simulink model "test_motor_2016a"  (R2016a)
settings: Solver=ode45  StartTime=0.0  StopTime=0.5  RelTol=1e-3
settings Model: Creator=Matias  LastModifiedBy=tomej
settings DataIOCC: SaveFormat=Structure

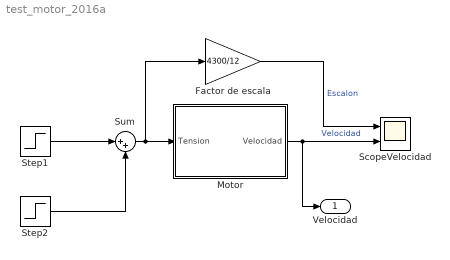
== system test_motor_2016a ==
  Factor de escala : Gain  Gain=4300/12
  Motor : Subsystem
  ScopeVelocidad : Scope  NumInputPorts=2
  Step1 : Step  Time=0  After=6  SampleTime=0
  Step2 : Step  Time=0.25  After=6  SampleTime=0
  Sum : Sum  Inputs=|++
  Velocidad : Outport
  wires:
  Step1/1 -> Sum/1
  Step2/1 -> Sum/2
  Motor/1(Velocidad) -> ScopeVelocidad/2, Velocidad/1  "Velocidad"
  Sum/1 -> Factor de escala/1, Motor/1(Tension)
  Factor de escala/1 -> ScopeVelocidad/1  "Escalon"

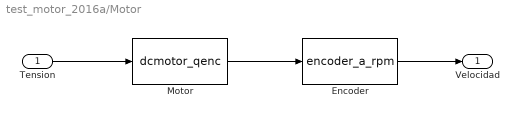
== system test_motor_2016a/Motor ==
  Tension : Inport
  Encoder : S-Function  FunctionName=encoder_a_rpm  Parameters=0.00001, 0.005,150  SFunctionDeploymentMode=off  EnableBusSupport=off
  Motor : S-Function  FunctionName=dcmotor_qenc  Parameters=150  SFunctionDeploymentMode=off  EnableBusSupport=off
  Velocidad : Outport
  wires:
  Motor/1 -> Encoder/1
  Encoder/1 -> Velocidad/1
  Tension/1 -> Motor/1
